simulink model "Mdl_11_OpenLoop"  (R2018a)
settings: Solver=VariableStepAuto  StartTime=0.0  StopTime=10.0  RelTol=1e-3
undefined symbols (not defined in the file): A_mdl, B_mdl, C_mdl, D_mdl, simSwitch
settings Model: Creator=pala  LastModifiedBy=pala
settings DataIOCC: SaveFinalState=on  SaveFormat=StructureWithTime  SaveState=on  SignalLogging=off  DSMLogging=off

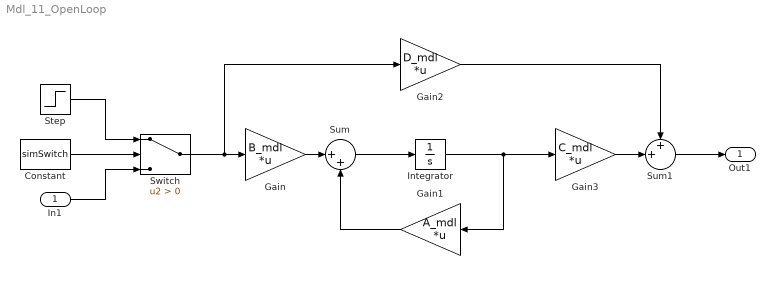
== system Mdl_11_OpenLoop ==
  In1 : Inport
  Constant : Constant  Value=simSwitch
  Gain : Gain  Gain=B_mdl  Multiplication=Matrix(K*u)
  Gain1 : Gain  Gain=A_mdl  Multiplication=Matrix(K*u)
  Gain2 : Gain  Gain=D_mdl  Multiplication=Matrix(K*u)
  Gain3 : Gain  Gain=C_mdl  Multiplication=Matrix(K*u)
  Integrator : Integrator
  Step : Step  SampleTime=0
  Sum : Sum  Inputs=|++
  Sum1 : Sum  Inputs=++|
  Switch : Switch  Criteria=u2 > Threshold
  Out1 : Outport
  wires:
  Step/1 -> Switch/1
  In1/1 -> Switch/3
  Constant/1 -> Switch/2
  Switch/1 -> Gain2/1, Gain/1
  Gain/1 -> Sum/1
  Gain1/1 -> Sum/2
  Sum/1 -> Integrator/1
  Integrator/1 -> Gain1/1, Gain3/1
  Gain2/1 -> Sum1/1
  Gain3/1 -> Sum1/2
  Sum1/1 -> Out1/1
